simulink model "Beautiful_powertrain"  (R2024a)
settings: Solver=ode3  StartTime=0.0  StopTime=40  FixedStep=0.001  RelTol=1e-3
model workspace (MAT data in the model file):
  C_Aero_drag = 0.28
  C_rolling_resistance = 0.01
  C_rolling_resitance = 0.01
  C_viscous_damping = 0.02
  Damping_coef = 50
  Gear_ratio = 10
  J_vehicle = 2.56328
  Motor_no_load_speed = 16000
  Motor_rated_load = 150000
  Motor_rated_speed = 9000
  Motor_rotor_damping = 0.02
  Motor_rotor_inertia = 0.05
  Motor_voltage = 450
  Slope = 0
  Vehicle_Wheel_Radius = 0.358
  Vehicle_frontal_area = 2.56
  Vehicle_mass = 2000
values from neighbouring files (symbols this model uses):
  s = sprintf('    [N_diangostic_2.m]
undefined symbols (not defined in the file or in its folder): battery_builder_rtmsupport, gcbh
libraries: Batteries_lib x36, fl_lib x31, nesl_utility x24, ee_lib x3, autolibshared x2, rllib x2, sdl_lib x1
(part 3 of 6)

== system Beautiful_powertrain/Motor ==
  Acc_cmd : Inport
  Brake_cmd : Inport  Port=2
  Controlled PWM Voltage : ee_lib/Integrated Circuits/Controlled PWM Voltage  F=1000 Hz  TD=0 s  pulse_width_offset=0 s  pulse_min=0 s  pwm_or_av=ee.enum.pwm_or_av.pwm  event_type=ee.enum.ic.event.asynchronous  sample_time=1e-6 s  Vmin=0 V  Vmax=1 V  Vm=5 V  u_min=0  u_max=1
  Controlled Voltage Source1 : fl_lib/Electrical/Electrical Sources/Controlled Voltage Source
  Controlled Voltage Source3 : fl_lib/Electrical/Electrical Sources/Controlled Voltage Source
  Current Sensor : fl_lib/Electrical/Electrical Sensors/Current Sensor
  DC Motor : ee_lib/Electromechanical/Brushed Motors/DC Motor  field_option=ee.enum.field_option.pm  Rf=100 Ohm  Lf=1 H  Laf=0.15 H  If0=0 A  parameterization=ee.enum.dcparam_option.load_speed  Ra=0.0093 Ohm  La=10 mH  emf_or_torque=ee.enum.emf_or_torque.kv  Kv=0.19 V/rpm  Ki=6.876e-4 N*m/A  T_stall=330 N*m  w_max=Motor_no_load_speed rpm  w_rated=Motor_rated_speed rpm  P_rated=Motor_rated_load kW  V_rated=Motor_voltage V  lam_param=ee.enum.lam_param.damping  i_noload=0 A  V_i_noload=1.5 V  J=Motor_rotor_inertia kg*m^2  lam=0 N*m*s/rad  speed0=0 rpm  enable_fault_armature=simscape.enum.onoff.off  rev_faulted=1 / 3  G_faulted_armature=1e-5 S  fault_trigger_armature=ee.enum.faults.faultTrigger.temporal  t_fault_armature=1 s  max_permissible_current_armature=inf A  t_fail_on_current_armature=1 s  enable_fault_field=simscape.enum.onoff.off  G_faulted_field=1e-5 S  fault_trigger_field=ee.enum.faults.faultTrigger.temporal  t_fault_field=1 s  max_permissible_current_field=inf A  t_fail_on_current_field=1 s  fault_action=simscape.enum.assert.action.none  alpha=3.93e-3 1/K  Tmeas=25 degC  thermal_mass=100 J/K  initial_temperature=25 degC
  Electrical Reference5 : fl_lib/Electrical/Electrical Elements/Electrical Reference
  Gain1 : Gain  Gain=1e-3
  H-Bridge : ee_lib/Semiconductors & Converters/Converters/H-Bridge  supply_ports=ee.enum.supply_ports.hidesupply  pwm_or_av=ee.enum.pwm_or_av.averaged  regenerative_braking_mode=ee.enum.converters.regenerative_braking_mode.always_enabled  discontinuous=ee.enum.current_profile.continuous  freewheeling_mode=ee.enum.converters.freewheeling_mode.one_switch_one_diode  Rload=10 Ohm  Lload=1e-5 H  F=10 kHz  Venable=2.5 V  Vmax=5 V  Vreverse=2.5 V  Vbrake=2.5 V  Vm=Motor_voltage V  Ron=0.1 Ohm  Don=0.05 Ohm  Goff=1e-6 S  Tmeas=298.15 K  Ron2=0.1 Ohm  Don2=0.05 Ohm  Tmeas2=398.15 K  thermal_mass=100 J/K  initial_temperature=298.15 K
  Mechanical Rotational Reference : fl_lib/Mechanical/Rotational Elements/Mechanical Rotational Reference
  PS-Simulink Converter : nesl_utility/PS-Simulink Converter  PhysicalDomain=network_engine_domain  SubClassName=ps_output  LeftPortType=input  RightPortType=output  PseudoPeriodic=off  Frequencies=[]  VectorFormat=inherit  Unit=inherit  AffineConversion=off
  PS-Simulink Converter1 : nesl_utility/PS-Simulink Converter  PhysicalDomain=network_engine_domain  SubClassName=ps_output  LeftPortType=input  RightPortType=output  PseudoPeriodic=off  Frequencies=[]  VectorFormat=inherit  Unit=inherit  AffineConversion=off
  Product : Product
  Simulink-PS Converter1 : nesl_utility/Simulink-PS Converter  PhysicalDomain=network_engine_domain  SubClassName=ps_input  LeftPortType=input  RightPortType=output  PseudoPeriodic=off  Frequencies=[]  NoiseDistribution=none  NoiseParameters=[]  Unit=1  AffineConversion=off  FilteringAndDerivatives=provide  SimscapeFilterOrder=1  InputFilterTimeConstant=0.001  UdotUserProvided=0
  Simulink-PS Converter2 : nesl_utility/Simulink-PS Converter  PhysicalDomain=network_engine_domain  SubClassName=ps_input  LeftPortType=input  RightPortType=output  PseudoPeriodic=off  Frequencies=[]  NoiseDistribution=none  NoiseParameters=[]  Unit=1  AffineConversion=off  FilteringAndDerivatives=provide  SimscapeFilterOrder=1  InputFilterTimeConstant=0.001  UdotUserProvided=0
  Solver Configuration2 : nesl_utility/Solver Configuration  PhysicalDomain=network_engine_domain  SubClassName=solver  LeftPortType=input  RightPortType=generic  Tones=[]  Harmonics=[]  SimulateNoise=off  Profile=off  UseLocalSampling=off  EnableSwitchedLinearOptims=on  FrequencyDomain=off  UseCCode=off  RelTol=0.001  AbsTol=0.001  MinStep=1e-09  ToWorkspace=off  RevertToSquareIcSolve=off  NumHomotopyIterations=100  PhasorMode=off  PhasorModeNumHarmonics=1  ConsistencySolver=NEWTON_XTOL_AFTER_FTOL  IndexReductionMethod=DerivativeReplacement  DoDC=off  ResidualTolerance=1e-09  ConsistencyTolSource=GLOBAL  ConsistencyAbsTol=0.001  ConsistencyRelTol=0.001  ConsistencyTolFactor=0.001  UseLocalSolver=off  LocalSolverChoice=NE_BACKWARD_EULER_ADVANCER  ResolveIndetEquations=on  FunctionEvalNumThread=1  LocalSolverSampleTime=0.001  DoFixedCost=off  MaxNonlinIter=3  MaxModeIter=2  ComputeImpulses=off  ImpulseIterations=2  LinearAlgebra=auto  LinearAlgebraNumThread=0  EquationFormulation=NE_TIME_EF  DelaysMemoryBudget=1024  AutomaticFiltering=on  FilteringTimeConstant=0.001  PartitionStorageMethod=AS_NEEDED  PartitionMemoryBudget=1024  PartitionMethod=ROBUST  MultibodyUseLocalSolver=off  MultibodyLocalSolverChoice=ODE1  MultibodyLocalSolverSampleTime=0.001
  To Workspace : ToWorkspace  VariableName=Motor_power  SaveFormat=Timeseries  SampleTime=-1
  Transfer Fcn : TransferFcn  Denominator=[1e-2 1]
  Voltage Sensor : fl_lib/Electrical/Electrical Sensors/Voltage Sensor
  Motor_current : PMIOPort  Side=Right
  Torque : PMIOPort  Port=2  Side=Right
  Ground : PMIOPort  Port=3  Side=Right
  wires:
  Acc_cmd/1 -> Simulink-PS Converter1/1
  Brake_cmd/1 -> Simulink-PS Converter2/1
  PS-Simulink Converter1/1 -> Product/1  "Motor_I"
  Product/1 -> Gain1/1
  Gain1/1 -> To Workspace/1  "Motor_P"
  Transfer Fcn/1 -> Product/2  "Motor_V"
  PS-Simulink Converter/1 -> Transfer Fcn/1
  connections:
  Simulink-PS Converter1/RConn1 -- Controlled Voltage Source1/RConn1
  Controlled Voltage Source1/LConn1 -- Controlled PWM Voltage/LConn1
  Simulink-PS Converter2/RConn1 -- Controlled Voltage Source3/RConn1
  Current Sensor/RConn1 -- PS-Simulink Converter1/LConn1 -- Motor_current/RConn1
  DC Motor/LConn2 -- Torque/RConn1
  Ground/RConn1 -- DC Motor/RConn2 -- Mechanical Rotational Reference/LConn1
  Controlled Voltage Source3/LConn1 -- H-Bridge/LConn4
  DC Motor/LConn1 -- Current Sensor/RConn2
  Controlled PWM Voltage/RConn1 -- H-Bridge/LConn1
  Controlled PWM Voltage/RConn2 -- H-Bridge/LConn2 -- H-Bridge/LConn3 -- Solver Configuration2/RConn1 -- Controlled Voltage Source1/RConn2 -- Controlled PWM Voltage/LConn2 -- Voltage Sensor/RConn2 -- H-Bridge/RConn2 -- DC Motor/RConn1 -- Controlled Voltage Source3/RConn2 -- Electrical Reference5/LConn1
  PS-Simulink Converter/LConn1 -- Voltage Sensor/RConn1
  Voltage Sensor/LConn1 -- Current Sensor/LConn1 -- H-Bridge/RConn1

== system Beautiful_powertrain/Sensors ==
  Gain1 : Gain  Gain=Vehicle_Wheel_Radius
  Ideal Rotational Motion Sensor : fl_lib/Mechanical/Mechanical Sensors/Ideal Rotational Motion Sensor  reference=foundation.enum.MeasurementReference.difference  acceleration_port=false  velocity_port=true  position_port=true  wrap_angle=false  offset=0 rad
  Ideal Rotational Motion Sensor1 : fl_lib/Mechanical/Mechanical Sensors/Ideal Rotational Motion Sensor  reference=foundation.enum.MeasurementReference.difference  acceleration_port=false  velocity_port=true  position_port=true  wrap_angle=false  offset=0 rad
  Mechanical Rotational Reference2 : fl_lib/Mechanical/Rotational Elements/Mechanical Rotational Reference
  Mechanical Rotational Reference3 : fl_lib/Mechanical/Rotational Elements/Mechanical Rotational Reference
  PS-Simulink Converter1 : nesl_utility/PS-Simulink Converter  PhysicalDomain=network_engine_domain  SubClassName=ps_output  LeftPortType=input  RightPortType=output  PseudoPeriodic=off  Frequencies=[]  VectorFormat=inherit  Unit=inherit  AffineConversion=off
  PS-Simulink Converter2 : nesl_utility/PS-Simulink Converter  PhysicalDomain=network_engine_domain  SubClassName=ps_output  LeftPortType=input  RightPortType=output  PseudoPeriodic=off  Frequencies=[]  VectorFormat=inherit  Unit=inherit  AffineConversion=off
  PS-Simulink Converter3 : nesl_utility/PS-Simulink Converter  PhysicalDomain=network_engine_domain  SubClassName=ps_output  LeftPortType=input  RightPortType=output  PseudoPeriodic=off  Frequencies=[]  VectorFormat=inherit  Unit=inherit  AffineConversion=off
  To Workspace4 : ToWorkspace  VariableName=Veh_Vel  SaveFormat=Structure With Time  SampleTime=-1
  In : PMIOPort  Side=Left
  Out : PMIOPort  Port=2  Side=Left
  I : Outport
  O : Outport  Port=2
  ACC : Outport  Port=3
  wires:
  PS-Simulink Converter1/1 -> I/1  "Velocity_ref"
  PS-Simulink Converter2/1 -> Gain1/1  "Output"
  Gain1/1 -> To Workspace4/1, O/1
  PS-Simulink Converter3/1 -> ACC/1  "Output"
  connections:
  Ideal Rotational Motion Sensor1/RConn3 -- PS-Simulink Converter3/LConn1
  PS-Simulink Converter1/LConn1 -- Ideal Rotational Motion Sensor/RConn2
  Ideal Rotational Motion Sensor/LConn1 -- In/RConn1
  Mechanical Rotational Reference3/LConn1 -- Ideal Rotational Motion Sensor1/RConn1
  PS-Simulink Converter2/LConn1 -- Ideal Rotational Motion Sensor1/RConn2
  Ideal Rotational Motion Sensor1/LConn1 -- Out/RConn1
  Ideal Rotational Motion Sensor/RConn1 -- Mechanical Rotational Reference2/LConn1

== system Beautiful_powertrain/Vel reference ==
  Constant1 : Constant
  Drive Cycle Source : autolibshared/Drive Cycle Source  cycleVar=FTP75  fileVar=cycleFTP75.mat  tfinal="2474  seconds"  cycleRepeat=off  outAccPort=off  outGearPort=off  gearList=No gear data  t_wot1=5  xdot_woto=0  xdot_wot1=30  t_wot2=20  xdot_wot2=0  t_wotend=30  srcUnit=m/s  outUnit=m/s  srcAccUnit=m/s/s  outAccUnit=m/s^2  dt=0  aMode=1  faultOption=off  velBnd=2  velBndUnit=mph  inUnit=m/s  timeBnd=1  failOption=off  stopSim=off  maxFaultCnt=10  maxFaultTime=2  maxTotFaultTime=15  traceOption=off  dtTrace=1  traceWindow=10  lastDCname=FTP75  lastOutUnit=mph  lastDT=0  lastTB=1  lastSB=2  forceCalcBound=off
  Multiport Switch : MultiPortSwitch  Inputs=4  SaturateOnIntegerOverflow=off  InputSameDT=off
  Pulse Generator : DiscretePulseGenerator  PulseType=Time based  Amplitude=5  Period=4  PulseWidth=50
  Sine Wave : Sin  Bias=1  Frequency=0.1  SampleTime=0
  Step : Step  After=13.9  SampleTime=0
  Step1 : Step  After=-13.9  SampleTime=0
  Sum1 : Sum  Inputs=|+-
  To Workspace5 : ToWorkspace  VariableName=Veh_ref  SaveFormat=Structure With Time  SampleTime=-1
  Vel_ref : Outport
  wires:
  Step/1 -> Sum1/1
  Multiport Switch/1 -> To Workspace5/1, Vel_ref/1  "Vel_ref"
  Drive Cycle Source/1 -> Multiport Switch/2
  Pulse Generator/1 -> Multiport Switch/4
  Step1/1 -> Sum1/2
  Sum1/1 -> Multiport Switch/3
  Constant1/1 -> Multiport Switch/1
  Sine Wave/1 -> Multiport Switch/5

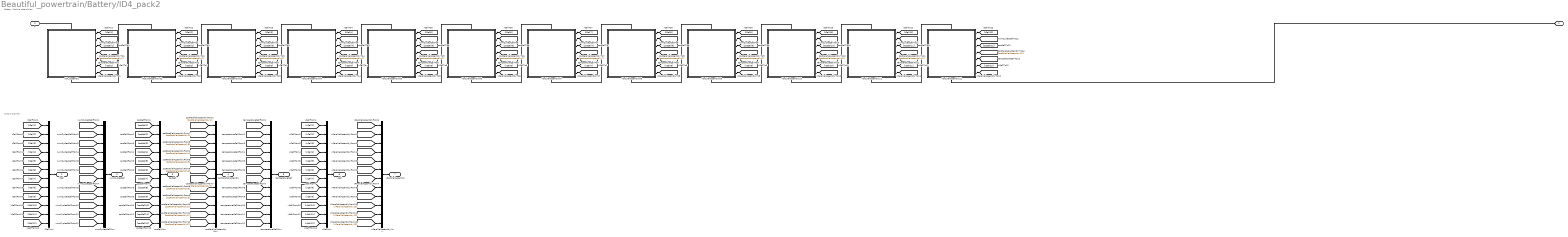
== system Beautiful_powertrain/Battery/ID4_pack2 ==
  note: Output Signals
  note: Battery Module Assemblies
  ID4_Assembly : Subsystem  LoadFcn=battery_builder_rtmsupport('loadfcn',gcbh);
      settings: CopyFcn=battery_builder_rtmsupport('copyfcn',gcbh);  PreCopyFcn=battery_builder_rtmsupport('precopyfcn',gcbh);  PreDeleteFcn=battery_builder_rtmsupport('predeletefcn',gcbh);  PortSchema="{\"entries\":[{\"content\":{\"sides\":[{\"content\":{\"connectorIds\":[\"LConn1\"]},\"type\":\"ConnectorPlacement.EquallySpacedRectSide\",\"uuid\":\"ff832d46-24c2-48f3-9ca2-acbc79ffea0e\"},{\"content\":{\"connectorIds\":[\"RConn1\"],\"side\":\"RIGHT\"},\"type\":\"ConnectorPlacement.EquallySpacedRectSide\",\"uuid\":\"f1f3b13c-36d9-4e7c-bb66-ad6aba201785\"},{\"content\":{\"side\":\"TOP\"},\"type\":\"ConnectorPlacement.EquallySpacedRectSide\",\"uuid\":\"497ed55c-0d21-4aaa-b04e-04d199c99403\"},{\"content\":{\"connectorIds\":[\"Out1\",\"Out2\",\"Out3\",\"Out4\",\"Out5\",\"Out6\",\"Out7\"],\"side\":\"BOTTOM\"},\"type\":\"ConnectorPlacement.EquallySpacedRectSide\",\"uuid\":\"076cd1de-5daa-42e2-9426-d52e4d178271\"}]},\"type\":\"ConnectorPlacement.EquallySpacedConnector\",\"uuid\":\"b44e404e-c709-4efd-83da-0fbfd4cccfd0\"}],\"packageUris\":[\"http://schema.mathworks.com/mf0/Connector/R2020b\"],\"version\":\"1.0\"}"
      mask Display: image('$imagefile')
  ModuleAssembly02 : Subsystem  LoadFcn=battery_builder_rtmsupport('loadfcn',gcbh);
      settings: CopyFcn=battery_builder_rtmsupport('copyfcn',gcbh);  PreCopyFcn=battery_builder_rtmsupport('precopyfcn',gcbh);  PreDeleteFcn=battery_builder_rtmsupport('predeletefcn',gcbh);  PortSchema="{\"entries\":[{\"content\":{\"sides\":[{\"content\":{\"connectorIds\":[\"LConn1\"]},\"type\":\"ConnectorPlacement.EquallySpacedRectSide\",\"uuid\":\"ff832d46-24c2-48f3-9ca2-acbc79ffea0e\"},{\"content\":{\"connectorIds\":[\"RConn1\"],\"side\":\"RIGHT\"},\"type\":\"ConnectorPlacement.EquallySpacedRectSide\",\"uuid\":\"f1f3b13c-36d9-4e7c-bb66-ad6aba201785\"},{\"content\":{\"side\":\"TOP\"},\"type\":\"ConnectorPlacement.EquallySpacedRectSide\",\"uuid\":\"497ed55c-0d21-4aaa-b04e-04d199c99403\"},{\"content\":{\"connectorIds\":[\"Out1\",\"Out2\",\"Out3\",\"Out4\",\"Out5\",\"Out6\",\"Out7\"],\"side\":\"BOTTOM\"},\"type\":\"ConnectorPlacement.EquallySpacedRectSide\",\"uuid\":\"076cd1de-5daa-42e2-9426-d52e4d178271\"}]},\"type\":\"ConnectorPlacement.EquallySpacedConnector\",\"uuid\":\"b44e404e-c709-4efd-83da-0fbfd4cccfd0\"}],\"packageUris\":[\"http://schema.mathworks.com/mf0/Connector/R2020b\"],\"version\":\"1.0\"}"
      mask Display: image('$imagefile')
  ModuleAssembly03 : Subsystem  LoadFcn=battery_builder_rtmsupport('loadfcn',gcbh);
      settings: CopyFcn=battery_builder_rtmsupport('copyfcn',gcbh);  PreCopyFcn=battery_builder_rtmsupport('precopyfcn',gcbh);  PreDeleteFcn=battery_builder_rtmsupport('predeletefcn',gcbh);  PortSchema="{\"entries\":[{\"content\":{\"sides\":[{\"content\":{\"connectorIds\":[\"LConn1\"]},\"type\":\"ConnectorPlacement.EquallySpacedRectSide\",\"uuid\":\"ff832d46-24c2-48f3-9ca2-acbc79ffea0e\"},{\"content\":{\"connectorIds\":[\"RConn1\"],\"side\":\"RIGHT\"},\"type\":\"ConnectorPlacement.EquallySpacedRectSide\",\"uuid\":\"f1f3b13c-36d9-4e7c-bb66-ad6aba201785\"},{\"content\":{\"side\":\"TOP\"},\"type\":\"ConnectorPlacement.EquallySpacedRectSide\",\"uuid\":\"497ed55c-0d21-4aaa-b04e-04d199c99403\"},{\"content\":{\"connectorIds\":[\"Out1\",\"Out2\",\"Out3\",\"Out4\",\"Out5\",\"Out6\",\"Out7\"],\"side\":\"BOTTOM\"},\"type\":\"ConnectorPlacement.EquallySpacedRectSide\",\"uuid\":\"076cd1de-5daa-42e2-9426-d52e4d178271\"}]},\"type\":\"ConnectorPlacement.EquallySpacedConnector\",\"uuid\":\"b44e404e-c709-4efd-83da-0fbfd4cccfd0\"}],\"packageUris\":[\"http://schema.mathworks.com/mf0/Connector/R2020b\"],\"version\":\"1.0\"}"
      mask Display: image('$imagefile')
  ModuleAssembly04 : Subsystem  LoadFcn=battery_builder_rtmsupport('loadfcn',gcbh);
      settings: CopyFcn=battery_builder_rtmsupport('copyfcn',gcbh);  PreCopyFcn=battery_builder_rtmsupport('precopyfcn',gcbh);  PreDeleteFcn=battery_builder_rtmsupport('predeletefcn',gcbh);  PortSchema="{\"entries\":[{\"content\":{\"sides\":[{\"content\":{\"connectorIds\":[\"LConn1\"]},\"type\":\"ConnectorPlacement.EquallySpacedRectSide\",\"uuid\":\"ff832d46-24c2-48f3-9ca2-acbc79ffea0e\"},{\"content\":{\"connectorIds\":[\"RConn1\"],\"side\":\"RIGHT\"},\"type\":\"ConnectorPlacement.EquallySpacedRectSide\",\"uuid\":\"f1f3b13c-36d9-4e7c-bb66-ad6aba201785\"},{\"content\":{\"side\":\"TOP\"},\"type\":\"ConnectorPlacement.EquallySpacedRectSide\",\"uuid\":\"497ed55c-0d21-4aaa-b04e-04d199c99403\"},{\"content\":{\"connectorIds\":[\"Out1\",\"Out2\",\"Out3\",\"Out4\",\"Out5\",\"Out6\",\"Out7\"],\"side\":\"BOTTOM\"},\"type\":\"ConnectorPlacement.EquallySpacedRectSide\",\"uuid\":\"076cd1de-5daa-42e2-9426-d52e4d178271\"}]},\"type\":\"ConnectorPlacement.EquallySpacedConnector\",\"uuid\":\"b44e404e-c709-4efd-83da-0fbfd4cccfd0\"}],\"packageUris\":[\"http://schema.mathworks.com/mf0/Connector/R2020b\"],\"version\":\"1.0\"}"
      mask Display: image('$imagefile')
  ModuleAssembly05 : Subsystem  LoadFcn=battery_builder_rtmsupport('loadfcn',gcbh);
      settings: CopyFcn=battery_builder_rtmsupport('copyfcn',gcbh);  PreCopyFcn=battery_builder_rtmsupport('precopyfcn',gcbh);  PreDeleteFcn=battery_builder_rtmsupport('predeletefcn',gcbh);  PortSchema="{\"entries\":[{\"content\":{\"sides\":[{\"content\":{\"connectorIds\":[\"LConn1\"]},\"type\":\"ConnectorPlacement.EquallySpacedRectSide\",\"uuid\":\"ff832d46-24c2-48f3-9ca2-acbc79ffea0e\"},{\"content\":{\"connectorIds\":[\"RConn1\"],\"side\":\"RIGHT\"},\"type\":\"ConnectorPlacement.EquallySpacedRectSide\",\"uuid\":\"f1f3b13c-36d9-4e7c-bb66-ad6aba201785\"},{\"content\":{\"side\":\"TOP\"},\"type\":\"ConnectorPlacement.EquallySpacedRectSide\",\"uuid\":\"497ed55c-0d21-4aaa-b04e-04d199c99403\"},{\"content\":{\"connectorIds\":[\"Out1\",\"Out2\",\"Out3\",\"Out4\",\"Out5\",\"Out6\",\"Out7\"],\"side\":\"BOTTOM\"},\"type\":\"ConnectorPlacement.EquallySpacedRectSide\",\"uuid\":\"076cd1de-5daa-42e2-9426-d52e4d178271\"}]},\"type\":\"ConnectorPlacement.EquallySpacedConnector\",\"uuid\":\"b44e404e-c709-4efd-83da-0fbfd4cccfd0\"}],\"packageUris\":[\"http://schema.mathworks.com/mf0/Connector/R2020b\"],\"version\":\"1.0\"}"
      mask Display: image('$imagefile')
  ModuleAssembly06 : Subsystem  LoadFcn=battery_builder_rtmsupport('loadfcn',gcbh);
      settings: CopyFcn=battery_builder_rtmsupport('copyfcn',gcbh);  PreCopyFcn=battery_builder_rtmsupport('precopyfcn',gcbh);  PreDeleteFcn=battery_builder_rtmsupport('predeletefcn',gcbh);  PortSchema="{\"entries\":[{\"content\":{\"sides\":[{\"content\":{\"connectorIds\":[\"LConn1\"]},\"type\":\"ConnectorPlacement.EquallySpacedRectSide\",\"uuid\":\"ff832d46-24c2-48f3-9ca2-acbc79ffea0e\"},{\"content\":{\"connectorIds\":[\"RConn1\"],\"side\":\"RIGHT\"},\"type\":\"ConnectorPlacement.EquallySpacedRectSide\",\"uuid\":\"f1f3b13c-36d9-4e7c-bb66-ad6aba201785\"},{\"content\":{\"side\":\"TOP\"},\"type\":\"ConnectorPlacement.EquallySpacedRectSide\",\"uuid\":\"497ed55c-0d21-4aaa-b04e-04d199c99403\"},{\"content\":{\"connectorIds\":[\"Out1\",\"Out2\",\"Out3\",\"Out4\",\"Out5\",\"Out6\",\"Out7\"],\"side\":\"BOTTOM\"},\"type\":\"ConnectorPlacement.EquallySpacedRectSide\",\"uuid\":\"076cd1de-5daa-42e2-9426-d52e4d178271\"}]},\"type\":\"ConnectorPlacement.EquallySpacedConnector\",\"uuid\":\"b44e404e-c709-4efd-83da-0fbfd4cccfd0\"}],\"packageUris\":[\"http://schema.mathworks.com/mf0/Connector/R2020b\"],\"version\":\"1.0\"}"
      mask Display: image('$imagefile')
  ModuleAssembly07 : Subsystem  LoadFcn=battery_builder_rtmsupport('loadfcn',gcbh);
      settings: CopyFcn=battery_builder_rtmsupport('copyfcn',gcbh);  PreCopyFcn=battery_builder_rtmsupport('precopyfcn',gcbh);  PreDeleteFcn=battery_builder_rtmsupport('predeletefcn',gcbh);  PortSchema="{\"entries\":[{\"content\":{\"sides\":[{\"content\":{\"connectorIds\":[\"LConn1\"]},\"type\":\"ConnectorPlacement.EquallySpacedRectSide\",\"uuid\":\"ff832d46-24c2-48f3-9ca2-acbc79ffea0e\"},{\"content\":{\"connectorIds\":[\"RConn1\"],\"side\":\"RIGHT\"},\"type\":\"ConnectorPlacement.EquallySpacedRectSide\",\"uuid\":\"f1f3b13c-36d9-4e7c-bb66-ad6aba201785\"},{\"content\":{\"side\":\"TOP\"},\"type\":\"ConnectorPlacement.EquallySpacedRectSide\",\"uuid\":\"497ed55c-0d21-4aaa-b04e-04d199c99403\"},{\"content\":{\"connectorIds\":[\"Out1\",\"Out2\",\"Out3\",\"Out4\",\"Out5\",\"Out6\",\"Out7\"],\"side\":\"BOTTOM\"},\"type\":\"ConnectorPlacement.EquallySpacedRectSide\",\"uuid\":\"076cd1de-5daa-42e2-9426-d52e4d178271\"}]},\"type\":\"ConnectorPlacement.EquallySpacedConnector\",\"uuid\":\"b44e404e-c709-4efd-83da-0fbfd4cccfd0\"}],\"packageUris\":[\"http://schema.mathworks.com/mf0/Connector/R2020b\"],\"version\":\"1.0\"}"
      mask Display: image('$imagefile')
  ModuleAssembly08 : Subsystem  LoadFcn=battery_builder_rtmsupport('loadfcn',gcbh);
      settings: CopyFcn=battery_builder_rtmsupport('copyfcn',gcbh);  PreCopyFcn=battery_builder_rtmsupport('precopyfcn',gcbh);  PreDeleteFcn=battery_builder_rtmsupport('predeletefcn',gcbh);  PortSchema="{\"entries\":[{\"content\":{\"sides\":[{\"content\":{\"connectorIds\":[\"LConn1\"]},\"type\":\"ConnectorPlacement.EquallySpacedRectSide\",\"uuid\":\"ff832d46-24c2-48f3-9ca2-acbc79ffea0e\"},{\"content\":{\"connectorIds\":[\"RConn1\"],\"side\":\"RIGHT\"},\"type\":\"ConnectorPlacement.EquallySpacedRectSide\",\"uuid\":\"f1f3b13c-36d9-4e7c-bb66-ad6aba201785\"},{\"content\":{\"side\":\"TOP\"},\"type\":\"ConnectorPlacement.EquallySpacedRectSide\",\"uuid\":\"497ed55c-0d21-4aaa-b04e-04d199c99403\"},{\"content\":{\"connectorIds\":[\"Out1\",\"Out2\",\"Out3\",\"Out4\",\"Out5\",\"Out6\",\"Out7\"],\"side\":\"BOTTOM\"},\"type\":\"ConnectorPlacement.EquallySpacedRectSide\",\"uuid\":\"076cd1de-5daa-42e2-9426-d52e4d178271\"}]},\"type\":\"ConnectorPlacement.EquallySpacedConnector\",\"uuid\":\"b44e404e-c709-4efd-83da-0fbfd4cccfd0\"}],\"packageUris\":[\"http://schema.mathworks.com/mf0/Connector/R2020b\"],\"version\":\"1.0\"}"
      mask Display: image('$imagefile')
  ModuleAssembly09 : Subsystem  LoadFcn=battery_builder_rtmsupport('loadfcn',gcbh);
      settings: CopyFcn=battery_builder_rtmsupport('copyfcn',gcbh);  PreCopyFcn=battery_builder_rtmsupport('precopyfcn',gcbh);  PreDeleteFcn=battery_builder_rtmsupport('predeletefcn',gcbh);  PortSchema="{\"entries\":[{\"content\":{\"sides\":[{\"content\":{\"connectorIds\":[\"LConn1\"]},\"type\":\"ConnectorPlacement.EquallySpacedRectSide\",\"uuid\":\"ff832d46-24c2-48f3-9ca2-acbc79ffea0e\"},{\"content\":{\"connectorIds\":[\"RConn1\"],\"side\":\"RIGHT\"},\"type\":\"ConnectorPlacement.EquallySpacedRectSide\",\"uuid\":\"f1f3b13c-36d9-4e7c-bb66-ad6aba201785\"},{\"content\":{\"side\":\"TOP\"},\"type\":\"ConnectorPlacement.EquallySpacedRectSide\",\"uuid\":\"497ed55c-0d21-4aaa-b04e-04d199c99403\"},{\"content\":{\"connectorIds\":[\"Out1\",\"Out2\",\"Out3\",\"Out4\",\"Out5\",\"Out6\",\"Out7\"],\"side\":\"BOTTOM\"},\"type\":\"ConnectorPlacement.EquallySpacedRectSide\",\"uuid\":\"076cd1de-5daa-42e2-9426-d52e4d178271\"}]},\"type\":\"ConnectorPlacement.EquallySpacedConnector\",\"uuid\":\"b44e404e-c709-4efd-83da-0fbfd4cccfd0\"}],\"packageUris\":[\"http://schema.mathworks.com/mf0/Connector/R2020b\"],\"version\":\"1.0\"}"
      mask Display: image('$imagefile')
  ModuleAssembly10 : Subsystem  LoadFcn=battery_builder_rtmsupport('loadfcn',gcbh);
      settings: CopyFcn=battery_builder_rtmsupport('copyfcn',gcbh);  PreCopyFcn=battery_builder_rtmsupport('precopyfcn',gcbh);  PreDeleteFcn=battery_builder_rtmsupport('predeletefcn',gcbh);  PortSchema="{\"entries\":[{\"content\":{\"sides\":[{\"content\":{\"connectorIds\":[\"LConn1\"]},\"type\":\"ConnectorPlacement.EquallySpacedRectSide\",\"uuid\":\"ff832d46-24c2-48f3-9ca2-acbc79ffea0e\"},{\"content\":{\"connectorIds\":[\"RConn1\"],\"side\":\"RIGHT\"},\"type\":\"ConnectorPlacement.EquallySpacedRectSide\",\"uuid\":\"f1f3b13c-36d9-4e7c-bb66-ad6aba201785\"},{\"content\":{\"side\":\"TOP\"},\"type\":\"ConnectorPlacement.EquallySpacedRectSide\",\"uuid\":\"497ed55c-0d21-4aaa-b04e-04d199c99403\"},{\"content\":{\"connectorIds\":[\"Out1\",\"Out2\",\"Out3\",\"Out4\",\"Out5\",\"Out6\",\"Out7\"],\"side\":\"BOTTOM\"},\"type\":\"ConnectorPlacement.EquallySpacedRectSide\",\"uuid\":\"076cd1de-5daa-42e2-9426-d52e4d178271\"}]},\"type\":\"ConnectorPlacement.EquallySpacedConnector\",\"uuid\":\"b44e404e-c709-4efd-83da-0fbfd4cccfd0\"}],\"packageUris\":[\"http://schema.mathworks.com/mf0/Connector/R2020b\"],\"version\":\"1.0\"}"
      mask Display: image('$imagefile')
  ModuleAssembly11 : Subsystem  LoadFcn=battery_builder_rtmsupport('loadfcn',gcbh);
      settings: CopyFcn=battery_builder_rtmsupport('copyfcn',gcbh);  PreCopyFcn=battery_builder_rtmsupport('precopyfcn',gcbh);  PreDeleteFcn=battery_builder_rtmsupport('predeletefcn',gcbh);  PortSchema="{\"entries\":[{\"content\":{\"sides\":[{\"content\":{\"connectorIds\":[\"LConn1\"]},\"type\":\"ConnectorPlacement.EquallySpacedRectSide\",\"uuid\":\"ff832d46-24c2-48f3-9ca2-acbc79ffea0e\"},{\"content\":{\"connectorIds\":[\"RConn1\"],\"side\":\"RIGHT\"},\"type\":\"ConnectorPlacement.EquallySpacedRectSide\",\"uuid\":\"f1f3b13c-36d9-4e7c-bb66-ad6aba201785\"},{\"content\":{\"side\":\"TOP\"},\"type\":\"ConnectorPlacement.EquallySpacedRectSide\",\"uuid\":\"497ed55c-0d21-4aaa-b04e-04d199c99403\"},{\"content\":{\"connectorIds\":[\"Out1\",\"Out2\",\"Out3\",\"Out4\",\"Out5\",\"Out6\",\"Out7\"],\"side\":\"BOTTOM\"},\"type\":\"ConnectorPlacement.EquallySpacedRectSide\",\"uuid\":\"076cd1de-5daa-42e2-9426-d52e4d178271\"}]},\"type\":\"ConnectorPlacement.EquallySpacedConnector\",\"uuid\":\"b44e404e-c709-4efd-83da-0fbfd4cccfd0\"}],\"packageUris\":[\"http://schema.mathworks.com/mf0/Connector/R2020b\"],\"version\":\"1.0\"}"
      mask Display: image('$imagefile')
  ModuleAssembly12 : Subsystem  LoadFcn=battery_builder_rtmsupport('loadfcn',gcbh);
      settings: CopyFcn=battery_builder_rtmsupport('copyfcn',gcbh);  PreCopyFcn=battery_builder_rtmsupport('precopyfcn',gcbh);  PreDeleteFcn=battery_builder_rtmsupport('predeletefcn',gcbh);  PortSchema="{\"entries\":[{\"content\":{\"sides\":[{\"content\":{\"connectorIds\":[\"LConn1\"]},\"type\":\"ConnectorPlacement.EquallySpacedRectSide\",\"uuid\":\"ff832d46-24c2-48f3-9ca2-acbc79ffea0e\"},{\"content\":{\"connectorIds\":[\"RConn1\"],\"side\":\"RIGHT\"},\"type\":\"ConnectorPlacement.EquallySpacedRectSide\",\"uuid\":\"f1f3b13c-36d9-4e7c-bb66-ad6aba201785\"},{\"content\":{\"side\":\"TOP\"},\"type\":\"ConnectorPlacement.EquallySpacedRectSide\",\"uuid\":\"497ed55c-0d21-4aaa-b04e-04d199c99403\"},{\"content\":{\"connectorIds\":[\"Out1\",\"Out2\",\"Out3\",\"Out4\",\"Out5\",\"Out6\",\"Out7\"],\"side\":\"BOTTOM\"},\"type\":\"ConnectorPlacement.EquallySpacedRectSide\",\"uuid\":\"076cd1de-5daa-42e2-9426-d52e4d178271\"}]},\"type\":\"ConnectorPlacement.EquallySpacedConnector\",\"uuid\":\"b44e404e-c709-4efd-83da-0fbfd4cccfd0\"}],\"packageUris\":[\"http://schema.mathworks.com/mf0/Connector/R2020b\"],\"version\":\"1.0\"}"
      mask Display: image('$imagefile')
  iCellMux : Mux  Inputs=12
  numCyclesCellMux : Mux  Inputs=12
  socCellMux : Mux  Inputs=12
  socParallelAssemblyMux : Mux  Inputs=12
  temperatureCellMux : Mux  Inputs=12
  vCellMux : Mux  Inputs=12
  vParallelAssemblyMux : Mux  Inputs=12
  - : PMIOPort  Port=2  Side=Right
  + : PMIOPort  Port=2  Side=Left
  iCell : Outport
  numCyclesCell : Outport  Port=2
  socCell : Outport  Port=3
  socParallelAssembly : Outport  Port=4
  temperatureCell : Outport  Port=5
  vCell : Outport  Port=6
  vParallelAssembly : Outport  Port=7
  wires:
  [vParallelAssembly12] -> vParallelAssemblyMux/12
  ModuleAssembly12/7(vParallelAssembly) -> [vParallelAssembly12]
  [vCell12] -> vCellMux/12
  ModuleAssembly12/6(vCell) -> [vCell12]
  [temperatureCell12] -> temperatureCellMux/12
  ModuleAssembly12/5(temperatureCell) -> [temperatureCell12]
  [socParallelAssembly12] -> socParallelAssemblyMux/12
  ModuleAssembly12/4(socParallelAssembly) -> [socParallelAssembly12]
  [socCell12] -> socCellMux/12
  ModuleAssembly12/3(socCell) -> [socCell12]
  [numCyclesCell12] -> numCyclesCellMux/12
  ModuleAssembly12/2(numCyclesCell) -> [numCyclesCell12]
  [iCell12] -> iCellMux/12
  ModuleAssembly12/1(iCell) -> [iCell12]
  [vParallelAssembly11] -> vParallelAssemblyMux/11
  ModuleAssembly11/7(vParallelAssembly) -> [vParallelAssembly11]
  [vCell11] -> vCellMux/11
  ModuleAssembly11/6(vCell) -> [vCell11]
  [temperatureCell11] -> temperatureCellMux/11
  ModuleAssembly11/5(temperatureCell) -> [temperatureCell11]
  [socParallelAssembly11] -> socParallelAssemblyMux/11
  ModuleAssembly11/4(socParallelAssembly) -> [socParallelAssembly11]
  [socCell11] -> socCellMux/11
  ModuleAssembly11/3(socCell) -> [socCell11]
  [numCyclesCell11] -> numCyclesCellMux/11
  ModuleAssembly11/2(numCyclesCell) -> [numCyclesCell11]
  [iCell11] -> iCellMux/11
  ModuleAssembly11/1(iCell) -> [iCell11]
  [vParallelAssembly10] -> vParallelAssemblyMux/10
  ModuleAssembly10/7(vParallelAssembly) -> [vParallelAssembly10]
  [vCell10] -> vCellMux/10
  ModuleAssembly10/6(vCell) -> [vCell10]
  [temperatureCell10] -> temperatureCellMux/10
  ModuleAssembly10/5(temperatureCell) -> [temperatureCell10]
  [socParallelAssembly10] -> socParallelAssemblyMux/10
  ModuleAssembly10/4(socParallelAssembly) -> [socParallelAssembly10]
  [socCell10] -> socCellMux/10
  ModuleAssembly10/3(socCell) -> [socCell10]
  [numCyclesCell10] -> numCyclesCellMux/10
  ModuleAssembly10/2(numCyclesCell) -> [numCyclesCell10]
  [iCell10] -> iCellMux/10
  ModuleAssembly10/1(iCell) -> [iCell10]
  [vParallelAssembly9] -> vParallelAssemblyMux/9
  ModuleAssembly09/7(vParallelAssembly) -> [vParallelAssembly9]
  [vCell9] -> vCellMux/9
  ModuleAssembly09/6(vCell) -> [vCell9]
  [temperatureCell9] -> temperatureCellMux/9
  ModuleAssembly09/5(temperatureCell) -> [temperatureCell9]
  [socParallelAssembly9] -> socParallelAssemblyMux/9
  ModuleAssembly09/4(socParallelAssembly) -> [socParallelAssembly9]
  [socCell9] -> socCellMux/9
  ModuleAssembly09/3(socCell) -> [socCell9]
  [numCyclesCell9] -> numCyclesCellMux/9
  ModuleAssembly09/2(numCyclesCell) -> [numCyclesCell9]
  [iCell9] -> iCellMux/9
  ModuleAssembly09/1(iCell) -> [iCell9]
  [vParallelAssembly8] -> vParallelAssemblyMux/8
  ModuleAssembly08/7(vParallelAssembly) -> [vParallelAssembly8]
  [vCell8] -> vCellMux/8
  ModuleAssembly08/6(vCell) -> [vCell8]
  [temperatureCell8] -> temperatureCellMux/8
  ModuleAssembly08/5(temperatureCell) -> [temperatureCell8]
  [socParallelAssembly8] -> socParallelAssemblyMux/8
  ModuleAssembly08/4(socParallelAssembly) -> [socParallelAssembly8]
  [socCell8] -> socCellMux/8
  ModuleAssembly08/3(socCell) -> [socCell8]
  [numCyclesCell8] -> numCyclesCellMux/8
  ModuleAssembly08/2(numCyclesCell) -> [numCyclesCell8]
  [iCell8] -> iCellMux/8
  ModuleAssembly08/1(iCell) -> [iCell8]
  [vParallelAssembly7] -> vParallelAssemblyMux/7
  ModuleAssembly07/7(vParallelAssembly) -> [vParallelAssembly7]
  [vCell7] -> vCellMux/7
  ModuleAssembly07/6(vCell) -> [vCell7]
  [temperatureCell7] -> temperatureCellMux/7
  ModuleAssembly07/5(temperatureCell) -> [temperatureCell7]
  [socParallelAssembly7] -> socParallelAssemblyMux/7
  ModuleAssembly07/4(socParallelAssembly) -> [socParallelAssembly7]
  [socCell7] -> socCellMux/7
  ModuleAssembly07/3(socCell) -> [socCell7]
  [numCyclesCell7] -> numCyclesCellMux/7
  ModuleAssembly07/2(numCyclesCell) -> [numCyclesCell7]
  [iCell7] -> iCellMux/7
  ModuleAssembly07/1(iCell) -> [iCell7]
  [vParallelAssembly6] -> vParallelAssemblyMux/6
  ModuleAssembly06/7(vParallelAssembly) -> [vParallelAssembly6]
  [vCell6] -> vCellMux/6
  ModuleAssembly06/6(vCell) -> [vCell6]
  [temperatureCell6] -> temperatureCellMux/6
  ModuleAssembly06/5(temperatureCell) -> [temperatureCell6]
  [socParallelAssembly6] -> socParallelAssemblyMux/6
  ModuleAssembly06/4(socParallelAssembly) -> [socParallelAssembly6]
  [socCell6] -> socCellMux/6
  ModuleAssembly06/3(socCell) -> [socCell6]
  [numCyclesCell6] -> numCyclesCellMux/6
  ModuleAssembly06/2(numCyclesCell) -> [numCyclesCell6]
  [iCell6] -> iCellMux/6
  ModuleAssembly06/1(iCell) -> [iCell6]
  [vParallelAssembly5] -> vParallelAssemblyMux/5
  ModuleAssembly05/7(vParallelAssembly) -> [vParallelAssembly5]
  [vCell5] -> vCellMux/5
  ModuleAssembly05/6(vCell) -> [vCell5]
  [temperatureCell5] -> temperatureCellMux/5
  ModuleAssembly05/5(temperatureCell) -> [temperatureCell5]
  [socParallelAssembly5] -> socParallelAssemblyMux/5
  ModuleAssembly05/4(socParallelAssembly) -> [socParallelAssembly5]
  [socCell5] -> socCellMux/5
  ModuleAssembly05/3(socCell) -> [socCell5]
  [numCyclesCell5] -> numCyclesCellMux/5
  ModuleAssembly05/2(numCyclesCell) -> [numCyclesCell5]
  [iCell5] -> iCellMux/5
  ModuleAssembly05/1(iCell) -> [iCell5]
  [vParallelAssembly4] -> vParallelAssemblyMux/4
  ModuleAssembly04/7(vParallelAssembly) -> [vParallelAssembly4]
  [vCell4] -> vCellMux/4
  ModuleAssembly04/6(vCell) -> [vCell4]
  [temperatureCell4] -> temperatureCellMux/4
  ModuleAssembly04/5(temperatureCell) -> [temperatureCell4]
  [socParallelAssembly4] -> socParallelAssemblyMux/4
  ModuleAssembly04/4(socParallelAssembly) -> [socParallelAssembly4]
  [socCell4] -> socCellMux/4
  ModuleAssembly04/3(socCell) -> [socCell4]
  [numCyclesCell4] -> numCyclesCellMux/4
  ModuleAssembly04/2(numCyclesCell) -> [numCyclesCell4]
  [iCell4] -> iCellMux/4
  ModuleAssembly04/1(iCell) -> [iCell4]
  [vParallelAssembly3] -> vParallelAssemblyMux/3
  ModuleAssembly03/7(vParallelAssembly) -> [vParallelAssembly3]
  [vCell3] -> vCellMux/3
  ModuleAssembly03/6(vCell) -> [vCell3]
  [temperatureCell3] -> temperatureCellMux/3
  ModuleAssembly03/5(temperatureCell) -> [temperatureCell3]
  [socParallelAssembly3] -> socParallelAssemblyMux/3
  ModuleAssembly03/4(socParallelAssembly) -> [socParallelAssembly3]
  [socCell3] -> socCellMux/3
  ModuleAssembly03/3(socCell) -> [socCell3]
  [numCyclesCell3] -> numCyclesCellMux/3
  ModuleAssembly03/2(numCyclesCell) -> [numCyclesCell3]
  [iCell3] -> iCellMux/3
  ModuleAssembly03/1(iCell) -> [iCell3]
  [vParallelAssembly2] -> vParallelAssemblyMux/2
  ModuleAssembly02/7(vParallelAssembly) -> [vParallelAssembly2]
  [vCell2] -> vCellMux/2
  ModuleAssembly02/6(vCell) -> [vCell2]
  [temperatureCell2] -> temperatureCellMux/2
  ModuleAssembly02/5(temperatureCell) -> [temperatureCell2]
  [socParallelAssembly2] -> socParallelAssemblyMux/2
  ModuleAssembly02/4(socParallelAssembly) -> [socParallelAssembly2]
  [socCell2] -> socCellMux/2
  ModuleAssembly02/3(socCell) -> [socCell2]
  [numCyclesCell2] -> numCyclesCellMux/2
  ModuleAssembly02/2(numCyclesCell) -> [numCyclesCell2]
  [iCell2] -> iCellMux/2
  ModuleAssembly02/1(iCell) -> [iCell2]
  [vParallelAssembly1] -> vParallelAssemblyMux/1
  vParallelAssemblyMux/1 -> vParallelAssembly/1
  ID4_Assembly/7(vParallelAssembly) -> [vParallelAssembly1]
  [vCell1] -> vCellMux/1
  vCellMux/1 -> vCell/1
  ID4_Assembly/6(vCell) -> [vCell1]
  [temperatureCell1] -> temperatureCellMux/1
  temperatureCellMux/1 -> temperatureCell/1
  ID4_Assembly/5(temperatureCell) -> [temperatureCell1]
  [socParallelAssembly1] -> socParallelAssemblyMux/1
  socParallelAssemblyMux/1 -> socParallelAssembly/1
  ID4_Assembly/4(socParallelAssembly) -> [socParallelAssembly1]
  [socCell1] -> socCellMux/1
  socCellMux/1 -> socCell/1
  ID4_Assembly/3(socCell) -> [socCell1]
  [numCyclesCell1] -> numCyclesCellMux/1
  numCyclesCellMux/1 -> numCyclesCell/1
  ID4_Assembly/2(numCyclesCell) -> [numCyclesCell1]
  [iCell1] -> iCellMux/1
  iCellMux/1 -> iCell/1
  ID4_Assembly/1(iCell) -> [iCell1]
  connections:
  ModuleAssembly12/RConn1 -- -/RConn1
  ID4_Assembly/LConn1 -- +/RConn1
  ModuleAssembly12/LConn1 -- ModuleAssembly11/RConn1
  ModuleAssembly11/LConn1 -- ModuleAssembly10/RConn1
  ModuleAssembly10/LConn1 -- ModuleAssembly09/RConn1
  ModuleAssembly09/LConn1 -- ModuleAssembly08/RConn1
  ModuleAssembly08/LConn1 -- ModuleAssembly07/RConn1
  ModuleAssembly07/LConn1 -- ModuleAssembly06/RConn1
  ModuleAssembly06/LConn1 -- ModuleAssembly05/RConn1
  ModuleAssembly05/LConn1 -- ModuleAssembly04/RConn1
  ModuleAssembly04/LConn1 -- ModuleAssembly03/RConn1
  ModuleAssembly03/LConn1 -- ModuleAssembly02/RConn1
  ModuleAssembly02/LConn1 -- ID4_Assembly/RConn1

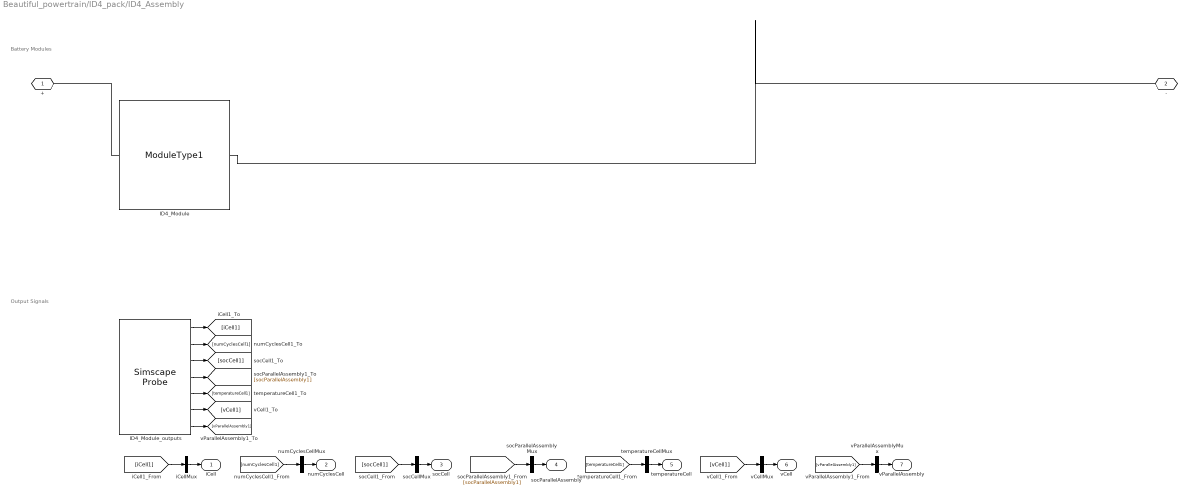
== system Beautiful_powertrain/ID4_pack/ID4_Assembly ==
  note: Battery Modules
  note: Output Signals
  ID4_Module : Batteries_lib/Modules/ModuleType1  SOC_vecCell=soc_vec  T_vecCell=T_vec K  V0_matCell=OCV_tbl V  V_rangeCell=V_range V  R0_matCell=R0_tbl Ohm  AHCell=Cap_Ah A*hr  extrapolation_optionCell=simscape.enum.extrapolation.nearest  thermal_massCell=100 J/K  P=3  S=8  iCell_specify=off  iCell_priority=None  iCell=0 A  iCell_nominal_specify=off  iCell_nominal_value=1  iCell_nominal_unit=A  vCell_specify=off  vCell_priority=None  vCell=0 V  vCell_nominal_specify=off  vCell_nominal_value=1  vCell_nominal_unit=V  socCell_specify=on  socCell_priority=High  socCell=SOC_start  socCell_nominal_specify=off  socCell_nominal_value=1  socCell_nominal_unit=1  numCyclesCell_specify=off  numCyclesCell_priority=High  numCyclesCell=0  numCyclesCell_nominal_specify=off  numCyclesCell_nominal_value=1  numCyclesCell_nominal_unit=1  temperatureCell_specify=off  temperatureCell_priority=High  temperatureCell=298.15 K  temperatureCell_nominal_specify=off  temperatureCell_nominal_value=1  temperatureCell_nominal_unit=K  vParallelAssembly_specify=off  vParallelAssembly_priority=None  vParallelAssembly=repmat(0, 8, 1) V  vParallelAssembly_nominal_specify=off  vParallelAssembly_nominal_value=1  vParallelAssembly_nominal_unit=V  socParallelAssembly_specify=off  socParallelAssembly_priority=None  socParallelAssembly=repmat(1, 8, 1)  socParallelAssembly_nominal_specify=off  socParallelAssembly_nominal_value=1  socParallelAssembly_nominal_unit=1
      settings: InternalSimscapePortConfiguration="{\"Bottom\":[{\"id\":\"n\",\"label\":\"-\",\"type\":\"foundation.electrical.electrical\"}],\"Left\":[],\"Right\":[],\"Top\":[{\"id\":\"p\",\"label\":\"+\",\"type\":\"foundation.electrical.electrical\"}]}"
  ID4_Module_outputs : SimscapeProbe  BoundBlock=330  Variables={iCell, numCyclesCell, socCell, socParallelAssembly, temperatureCell, vCell, vParallelAssembly}
  iCellMux : Mux  Inputs=1
  numCyclesCellMux : Mux  Inputs=1
  socCellMux : Mux  Inputs=1
  socParallelAssemblyMux : Mux  Inputs=1
  temperatureCellMux : Mux  Inputs=1
  vCellMux : Mux  Inputs=1
  vParallelAssemblyMux : Mux  Inputs=1
  + : PMIOPort  Side=Left
  - : PMIOPort  Port=2  Side=Right
  iCell : Outport
  numCyclesCell : Outport  Port=2
  socCell : Outport  Port=3
  socParallelAssembly : Outport  Port=4
  temperatureCell : Outport  Port=5
  vCell : Outport  Port=6
  vParallelAssembly : Outport  Port=7
  wires:
  ID4_Module_outputs/1 -> [iCell1]
  iCellMux/1 -> iCell/1
  [iCell1] -> iCellMux/1
  ID4_Module_outputs/2 -> [numCyclesCell1]
  numCyclesCellMux/1 -> numCyclesCell/1
  [numCyclesCell1] -> numCyclesCellMux/1
  ID4_Module_outputs/3 -> [socCell1]
  socCellMux/1 -> socCell/1
  [socCell1] -> socCellMux/1
  ID4_Module_outputs/4 -> [socParallelAssembly1]
  socParallelAssemblyMux/1 -> socParallelAssembly/1
  [socParallelAssembly1] -> socParallelAssemblyMux/1
  ID4_Module_outputs/5 -> [temperatureCell1]
  temperatureCellMux/1 -> temperatureCell/1
  [temperatureCell1] -> temperatureCellMux/1
  ID4_Module_outputs/6 -> [vCell1]
  vCellMux/1 -> vCell/1
  [vCell1] -> vCellMux/1
  ID4_Module_outputs/7 -> [vParallelAssembly1]
  vParallelAssemblyMux/1 -> vParallelAssembly/1
  [vParallelAssembly1] -> vParallelAssemblyMux/1
  connections:
  ID4_Module/LConn1 -- +/RConn1
  ID4_Module/RConn1 -- -/RConn1

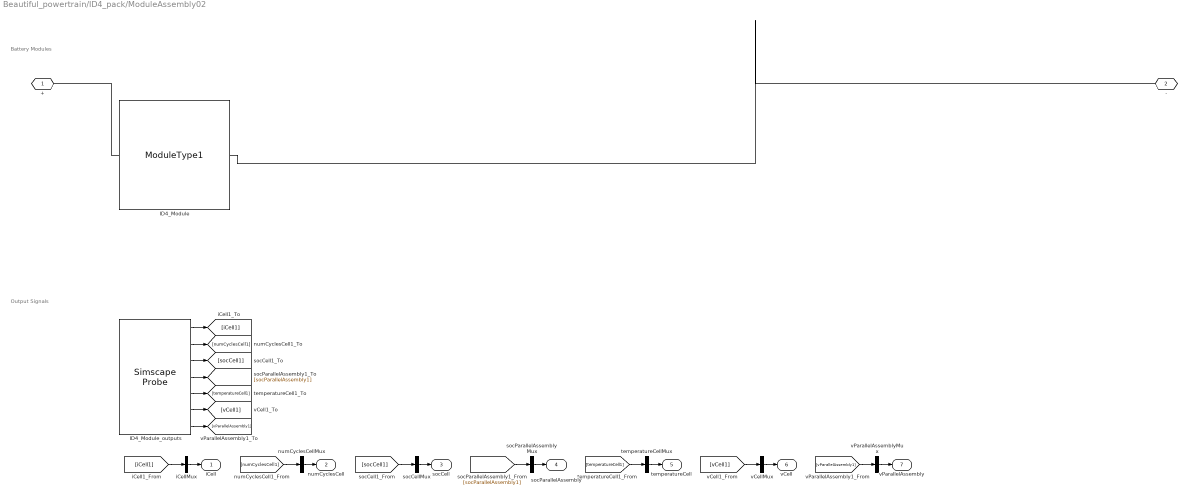
== system Beautiful_powertrain/ID4_pack/ModuleAssembly02 ==
  note: Battery Modules
  note: Output Signals
  ID4_Module : Batteries_lib/Modules/ModuleType1  SOC_vecCell=soc_vec  T_vecCell=T_vec K  V0_matCell=OCV_tbl V  V_rangeCell=V_range V  R0_matCell=R0_tbl Ohm  AHCell=Cap_Ah A*hr  extrapolation_optionCell=simscape.enum.extrapolation.nearest  thermal_massCell=100 J/K  P=3  S=8  iCell_specify=off  iCell_priority=None  iCell=0 A  iCell_nominal_specify=off  iCell_nominal_value=1  iCell_nominal_unit=A  vCell_specify=off  vCell_priority=None  vCell=0 V  vCell_nominal_specify=off  vCell_nominal_value=1  vCell_nominal_unit=V  socCell_specify=on  socCell_priority=High  socCell=SOC_start  socCell_nominal_specify=off  socCell_nominal_value=1  socCell_nominal_unit=1  numCyclesCell_specify=off  numCyclesCell_priority=High  numCyclesCell=0  numCyclesCell_nominal_specify=off  numCyclesCell_nominal_value=1  numCyclesCell_nominal_unit=1  temperatureCell_specify=off  temperatureCell_priority=High  temperatureCell=298.15 K  temperatureCell_nominal_specify=off  temperatureCell_nominal_value=1  temperatureCell_nominal_unit=K  vParallelAssembly_specify=off  vParallelAssembly_priority=None  vParallelAssembly=repmat(0, 8, 1) V  vParallelAssembly_nominal_specify=off  vParallelAssembly_nominal_value=1  vParallelAssembly_nominal_unit=V  socParallelAssembly_specify=off  socParallelAssembly_priority=None  socParallelAssembly=repmat(1, 8, 1)  socParallelAssembly_nominal_specify=off  socParallelAssembly_nominal_value=1  socParallelAssembly_nominal_unit=1
      settings: InternalSimscapePortConfiguration="{\"Bottom\":[{\"id\":\"n\",\"label\":\"-\",\"type\":\"foundation.electrical.electrical\"}],\"Left\":[],\"Right\":[],\"Top\":[{\"id\":\"p\",\"label\":\"+\",\"type\":\"foundation.electrical.electrical\"}]}"
  ID4_Module_outputs : SimscapeProbe  BoundBlock=365  Variables={iCell, numCyclesCell, socCell, socParallelAssembly, temperatureCell, vCell, vParallelAssembly}
  iCellMux : Mux  Inputs=1
  numCyclesCellMux : Mux  Inputs=1
  socCellMux : Mux  Inputs=1
  socParallelAssemblyMux : Mux  Inputs=1
  temperatureCellMux : Mux  Inputs=1
  vCellMux : Mux  Inputs=1
  vParallelAssemblyMux : Mux  Inputs=1
  + : PMIOPort  Side=Left
  - : PMIOPort  Port=2  Side=Right
  iCell : Outport
  numCyclesCell : Outport  Port=2
  socCell : Outport  Port=3
  socParallelAssembly : Outport  Port=4
  temperatureCell : Outport  Port=5
  vCell : Outport  Port=6
  vParallelAssembly : Outport  Port=7
  wires:
  ID4_Module_outputs/1 -> [iCell1]
  iCellMux/1 -> iCell/1
  [iCell1] -> iCellMux/1
  ID4_Module_outputs/2 -> [numCyclesCell1]
  numCyclesCellMux/1 -> numCyclesCell/1
  [numCyclesCell1] -> numCyclesCellMux/1
  ID4_Module_outputs/3 -> [socCell1]
  socCellMux/1 -> socCell/1
  [socCell1] -> socCellMux/1
  ID4_Module_outputs/4 -> [socParallelAssembly1]
  socParallelAssemblyMux/1 -> socParallelAssembly/1
  [socParallelAssembly1] -> socParallelAssemblyMux/1
  ID4_Module_outputs/5 -> [temperatureCell1]
  temperatureCellMux/1 -> temperatureCell/1
  [temperatureCell1] -> temperatureCellMux/1
  ID4_Module_outputs/6 -> [vCell1]
  vCellMux/1 -> vCell/1
  [vCell1] -> vCellMux/1
  ID4_Module_outputs/7 -> [vParallelAssembly1]
  vParallelAssemblyMux/1 -> vParallelAssembly/1
  [vParallelAssembly1] -> vParallelAssemblyMux/1
  connections:
  ID4_Module/LConn1 -- +/RConn1
  ID4_Module/RConn1 -- -/RConn1

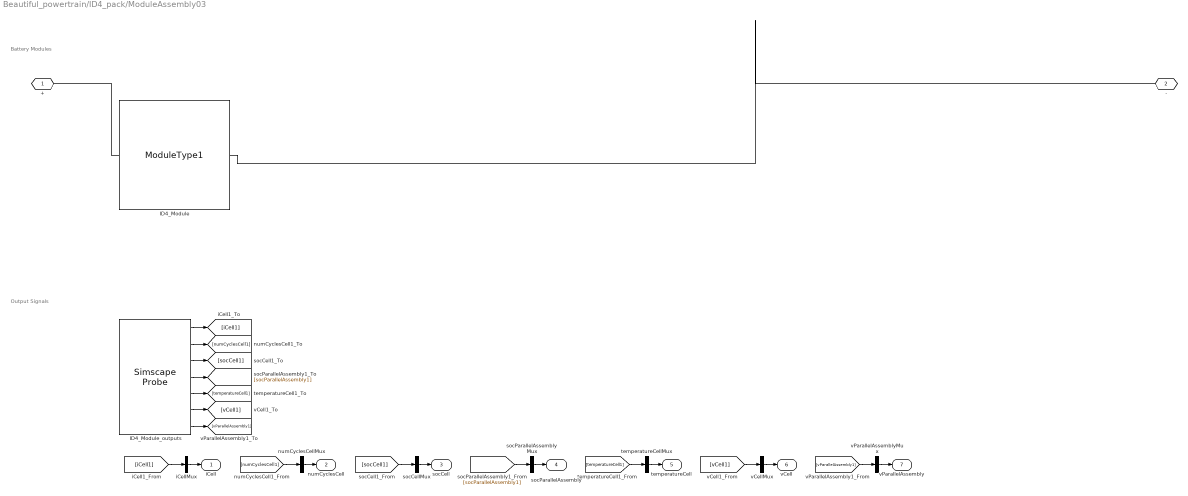
== system Beautiful_powertrain/ID4_pack/ModuleAssembly03 ==
  note: Battery Modules
  note: Output Signals
  ID4_Module : Batteries_lib/Modules/ModuleType1  SOC_vecCell=soc_vec  T_vecCell=T_vec K  V0_matCell=OCV_tbl V  V_rangeCell=V_range V  R0_matCell=R0_tbl Ohm  AHCell=Cap_Ah A*hr  extrapolation_optionCell=simscape.enum.extrapolation.nearest  thermal_massCell=100 J/K  P=3  S=8  iCell_specify=off  iCell_priority=None  iCell=0 A  iCell_nominal_specify=off  iCell_nominal_value=1  iCell_nominal_unit=A  vCell_specify=off  vCell_priority=None  vCell=0 V  vCell_nominal_specify=off  vCell_nominal_value=1  vCell_nominal_unit=V  socCell_specify=on  socCell_priority=High  socCell=SOC_start  socCell_nominal_specify=off  socCell_nominal_value=1  socCell_nominal_unit=1  numCyclesCell_specify=off  numCyclesCell_priority=High  numCyclesCell=0  numCyclesCell_nominal_specify=off  numCyclesCell_nominal_value=1  numCyclesCell_nominal_unit=1  temperatureCell_specify=off  temperatureCell_priority=High  temperatureCell=298.15 K  temperatureCell_nominal_specify=off  temperatureCell_nominal_value=1  temperatureCell_nominal_unit=K  vParallelAssembly_specify=off  vParallelAssembly_priority=None  vParallelAssembly=repmat(0, 8, 1) V  vParallelAssembly_nominal_specify=off  vParallelAssembly_nominal_value=1  vParallelAssembly_nominal_unit=V  socParallelAssembly_specify=off  socParallelAssembly_priority=None  socParallelAssembly=repmat(1, 8, 1)  socParallelAssembly_nominal_specify=off  socParallelAssembly_nominal_value=1  socParallelAssembly_nominal_unit=1
      settings: InternalSimscapePortConfiguration="{\"Bottom\":[{\"id\":\"n\",\"label\":\"-\",\"type\":\"foundation.electrical.electrical\"}],\"Left\":[],\"Right\":[],\"Top\":[{\"id\":\"p\",\"label\":\"+\",\"type\":\"foundation.electrical.electrical\"}]}"
  ID4_Module_outputs : SimscapeProbe  BoundBlock=400  Variables={iCell, numCyclesCell, socCell, socParallelAssembly, temperatureCell, vCell, vParallelAssembly}
  iCellMux : Mux  Inputs=1
  numCyclesCellMux : Mux  Inputs=1
  socCellMux : Mux  Inputs=1
  socParallelAssemblyMux : Mux  Inputs=1
  temperatureCellMux : Mux  Inputs=1
  vCellMux : Mux  Inputs=1
  vParallelAssemblyMux : Mux  Inputs=1
  + : PMIOPort  Side=Left
  - : PMIOPort  Port=2  Side=Right
  iCell : Outport
  numCyclesCell : Outport  Port=2
  socCell : Outport  Port=3
  socParallelAssembly : Outport  Port=4
  temperatureCell : Outport  Port=5
  vCell : Outport  Port=6
  vParallelAssembly : Outport  Port=7
  wires:
  ID4_Module_outputs/1 -> [iCell1]
  iCellMux/1 -> iCell/1
  [iCell1] -> iCellMux/1
  ID4_Module_outputs/2 -> [numCyclesCell1]
  numCyclesCellMux/1 -> numCyclesCell/1
  [numCyclesCell1] -> numCyclesCellMux/1
  ID4_Module_outputs/3 -> [socCell1]
  socCellMux/1 -> socCell/1
  [socCell1] -> socCellMux/1
  ID4_Module_outputs/4 -> [socParallelAssembly1]
  socParallelAssemblyMux/1 -> socParallelAssembly/1
  [socParallelAssembly1] -> socParallelAssemblyMux/1
  ID4_Module_outputs/5 -> [temperatureCell1]
  temperatureCellMux/1 -> temperatureCell/1
  [temperatureCell1] -> temperatureCellMux/1
  ID4_Module_outputs/6 -> [vCell1]
  vCellMux/1 -> vCell/1
  [vCell1] -> vCellMux/1
  ID4_Module_outputs/7 -> [vParallelAssembly1]
  vParallelAssemblyMux/1 -> vParallelAssembly/1
  [vParallelAssembly1] -> vParallelAssemblyMux/1
  connections:
  ID4_Module/LConn1 -- +/RConn1
  ID4_Module/RConn1 -- -/RConn1

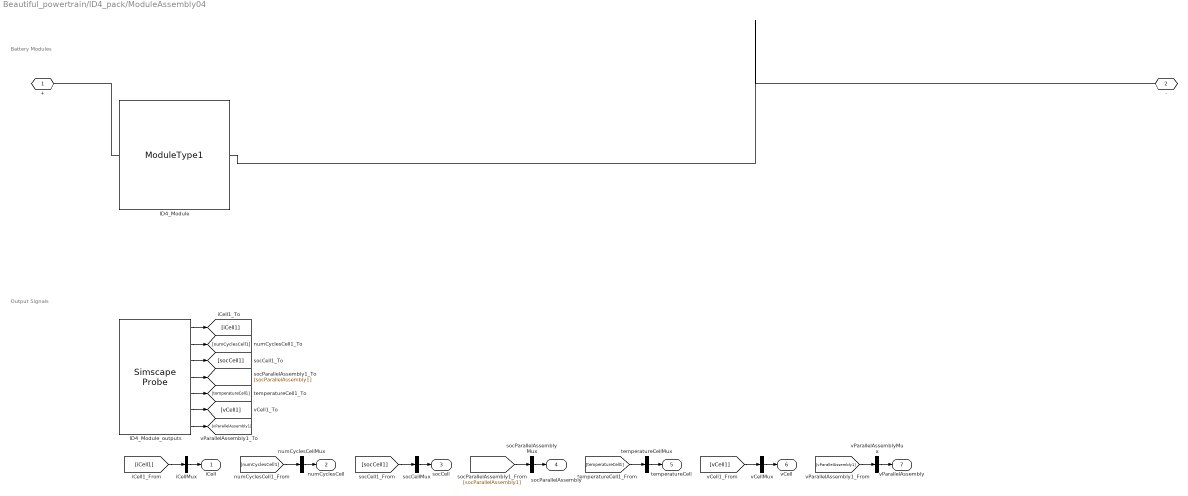
== system Beautiful_powertrain/ID4_pack/ModuleAssembly04 ==
  note: Battery Modules
  note: Output Signals
  ID4_Module : Batteries_lib/Modules/ModuleType1  SOC_vecCell=soc_vec  T_vecCell=T_vec K  V0_matCell=OCV_tbl V  V_rangeCell=V_range V  R0_matCell=R0_tbl Ohm  AHCell=Cap_Ah A*hr  extrapolation_optionCell=simscape.enum.extrapolation.nearest  thermal_massCell=100 J/K  P=3  S=8  iCell_specify=off  iCell_priority=None  iCell=0 A  iCell_nominal_specify=off  iCell_nominal_value=1  iCell_nominal_unit=A  vCell_specify=off  vCell_priority=None  vCell=0 V  vCell_nominal_specify=off  vCell_nominal_value=1  vCell_nominal_unit=V  socCell_specify=on  socCell_priority=High  socCell=SOC_start  socCell_nominal_specify=off  socCell_nominal_value=1  socCell_nominal_unit=1  numCyclesCell_specify=off  numCyclesCell_priority=High  numCyclesCell=0  numCyclesCell_nominal_specify=off  numCyclesCell_nominal_value=1  numCyclesCell_nominal_unit=1  temperatureCell_specify=off  temperatureCell_priority=High  temperatureCell=298.15 K  temperatureCell_nominal_specify=off  temperatureCell_nominal_value=1  temperatureCell_nominal_unit=K  vParallelAssembly_specify=off  vParallelAssembly_priority=None  vParallelAssembly=repmat(0, 8, 1) V  vParallelAssembly_nominal_specify=off  vParallelAssembly_nominal_value=1  vParallelAssembly_nominal_unit=V  socParallelAssembly_specify=off  socParallelAssembly_priority=None  socParallelAssembly=repmat(1, 8, 1)  socParallelAssembly_nominal_specify=off  socParallelAssembly_nominal_value=1  socParallelAssembly_nominal_unit=1
      settings: InternalSimscapePortConfiguration="{\"Bottom\":[{\"id\":\"n\",\"label\":\"-\",\"type\":\"foundation.electrical.electrical\"}],\"Left\":[],\"Right\":[],\"Top\":[{\"id\":\"p\",\"label\":\"+\",\"type\":\"foundation.electrical.electrical\"}]}"
  ID4_Module_outputs : SimscapeProbe  BoundBlock=435  Variables={iCell, numCyclesCell, socCell, socParallelAssembly, temperatureCell, vCell, vParallelAssembly}
  iCellMux : Mux  Inputs=1
  numCyclesCellMux : Mux  Inputs=1
  socCellMux : Mux  Inputs=1
  socParallelAssemblyMux : Mux  Inputs=1
  temperatureCellMux : Mux  Inputs=1
  vCellMux : Mux  Inputs=1
  vParallelAssemblyMux : Mux  Inputs=1
  + : PMIOPort  Side=Left
  - : PMIOPort  Port=2  Side=Right
  iCell : Outport
  numCyclesCell : Outport  Port=2
  socCell : Outport  Port=3
  socParallelAssembly : Outport  Port=4
  temperatureCell : Outport  Port=5
  vCell : Outport  Port=6
  vParallelAssembly : Outport  Port=7
  wires:
  ID4_Module_outputs/1 -> [iCell1]
  iCellMux/1 -> iCell/1
  [iCell1] -> iCellMux/1
  ID4_Module_outputs/2 -> [numCyclesCell1]
  numCyclesCellMux/1 -> numCyclesCell/1
  [numCyclesCell1] -> numCyclesCellMux/1
  ID4_Module_outputs/3 -> [socCell1]
  socCellMux/1 -> socCell/1
  [socCell1] -> socCellMux/1
  ID4_Module_outputs/4 -> [socParallelAssembly1]
  socParallelAssemblyMux/1 -> socParallelAssembly/1
  [socParallelAssembly1] -> socParallelAssemblyMux/1
  ID4_Module_outputs/5 -> [temperatureCell1]
  temperatureCellMux/1 -> temperatureCell/1
  [temperatureCell1] -> temperatureCellMux/1
  ID4_Module_outputs/6 -> [vCell1]
  vCellMux/1 -> vCell/1
  [vCell1] -> vCellMux/1
  ID4_Module_outputs/7 -> [vParallelAssembly1]
  vParallelAssemblyMux/1 -> vParallelAssembly/1
  [vParallelAssembly1] -> vParallelAssemblyMux/1
  connections:
  ID4_Module/LConn1 -- +/RConn1
  ID4_Module/RConn1 -- -/RConn1
